simulink library "pm_machines_library"  (R2016b)
settings: Solver=ode45  StartTime=0.0  StopTime=10.0  RelTol=1e-3  EnableMultiTasking=on
libraries: powerlib x9, pm_machines_library x4, powerlib_extras x3
settings Model: Creator=s0237326  LastModifiedBy=rcrozier
settings DataIOCC: LimitDataPoints=on  SaveFormat=Array  SignalLoggingSaveFormat=ModelDataLogs
settings OptimizationCC: ExpressionDepthLimit=2147483647  LifeSpan=inf
settings DebuggingCC: UnderspecifiedInitializationDetection=Classic  MergeDetectMultiDrivingBlocksExec=none  SolverPrmCheckMsg=warning  FcnCallInpInsideContextMsg=warning  StateNameClashWarn=warning  SFUnexpectedBacktrackingDiag=warning  SFNoUnconditionalDefaultTransitionDiag=warning  SFExecutionAtInitializationDiag=none
settings HardwareCC: ProdBitPerPointer=32  ProdBitPerSizeT=32  ProdBitPerPtrDiffT=32  ProdLargestAtomicFloat=None  ProdIntDivRoundTo=Undefined  ProdEndianess=Unspecified  ProdWordSize=32  ProdHWDeviceType=32-bit Generic
settings ModelReferenceCC: PropagateSignalLabelsOutOfModel=off
settings GRTTargetCC: TargetLangStandard=C89/C90 (ANSI)  GeneratePreprocessorConditionals=Disable all  CombineOutputUpdateFcns=off  GRTInterface=on
settings ConfigComp: CovMetricSettings=dw  CovHtmlReporting=on  CovSaveCumulativeToWorkspaceVar=on  CovSaveSingleToWorkspaceVar=on  CovExternalEMLEnable=off

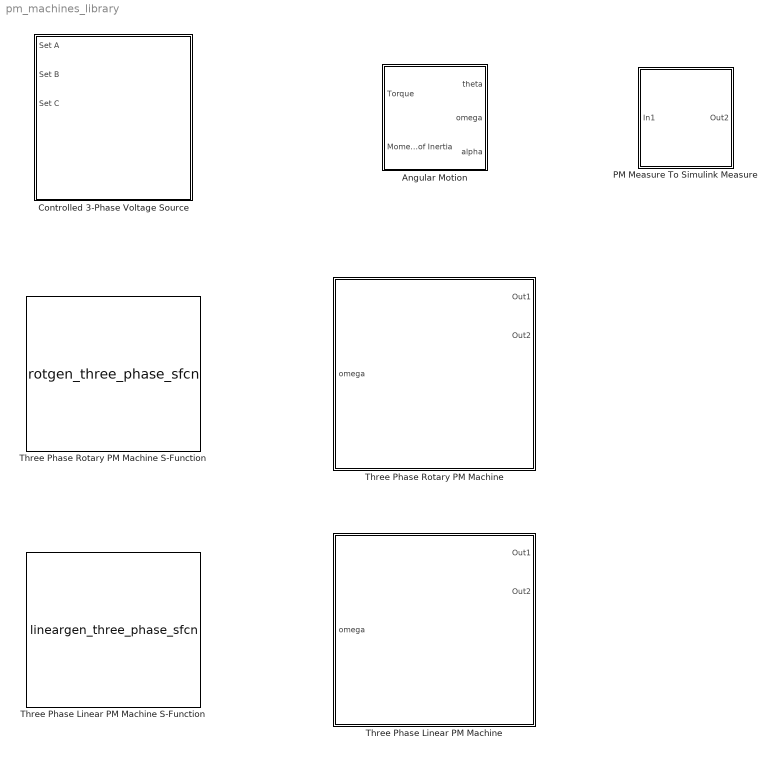
== system pm_machines_library ==
  Angular Motion : Subsystem
  Controlled 3-Phase Voltage Source : Subsystem  mask(Controlled 3-Phase Voltage Source){}
      mask help: Controlled 3-Phase Voltage Source Mask
      mask DialogControl DescGroupVar Prompt: Controlled Three Phase Voltage Source
      mask DialogControl DescTextVar Prompt: A block of three SimPowerSystems controlled voltage sources for interfacing non-SimPowerSystems three phase signals into SimPowerSystems simulations. Provided for convenience, used by other library blocks.
  PM Measure To Simulink Measure : Subsystem  mask{ref_type=Stationary}
      mask prompts: ref_type "dq Reference Type"
      mask TypeOptions ref_type: Synchronous | Stationary
      mask DialogControl DescTextVar Prompt: Converts the outputs of the PM Machines library blocks to the same format as the native simulink electrical machine models proide as 'measurements'.
  Three Phase Linear PM Machine : Subsystem  mask{design_data_type_popup=From File, file_name_edit=Enter file path here, design_workspace_edit=[], simoptions_workspace_edit=[]}
      mask prompts: design_data_type_popup "Design Data Type"; file_name_edit "File containing design and Simoptions data structures"; design_workspace_edit "Design structure variable in workspace"; simoptions_workspace_edit "Simoptions structure variable name"
      mask init:
      | data_ready = false;
      | 
      | if design_data_type_popup == 1
      |     
      |     if ~(strcmp(file_name_edit, 'Enter file path here') ...
      |             || isempty(file_name_edit))
      | 
      |         % get the file name
      |         design_data_file = file_name_edit;
      |         
      |         % check it exists
      |         if exist (design_data_file, 'file') == 2
      |             % check if right data is in file
      |             try
      |                 load (design_data_file, 'design', 'simoptions');
      |             catch ME
      |                 error ('RENEWNET:rotgen_three_phase_sfcn:badfile', ...
      |                 'Loading design data from file\n\n %s\n\nfailed with the following error message:\n\n"%s"\n\n', ...
      |                     design_data_file, ME.message);
      |             end
      |             
      |             data_ready = true;
      | 
      |         else
      |             error ('RENEWNET:rotgen_three_phase_sfcn:badfile', ...
      |                 'Design data file\n: %s\ndoes not appear to exist', design_data_file);
      |         end
      |     
      |     end
      | 
      | elseif design_data_type_popup == 2
      |     % get the variable names
      |     design = design_workspace_edit;
      |     simoptions = simoptions_workspace_edit;
      |     
      |     if ~isempty (design) && ~isempty (simoptions)
      |         data_ready = true;
      |     end
      | else
      |     error ('RENEWNET:rotgen_three_phase_sfcn:baddatatype', ...
      |         'Invalid Data Type popup value')
      | end
      | 
      | if data_ready
      |     
      |     % do some checks on the data
      |     if design.Phases ~= 3
      |         error('Design must have three Phases.')
      |     end
      | 
      |     if ~isfield(design, 'slm_fluxlinkage')
      |         error('Design data does not appear to be complete (no flux linage info)')
      |     end
      | 
      |     blk = gcb;                                         
      |     % set_param([gcb, '/adder1/Gain'],'Gain','A')
      | 
      |     set_param([blk, '/Windings'], 'SelfImpedance1', sprintf('[%f %f]', design.PhaseResistance(1), design.PhaseInductance(1)));
      |     set_param([blk, '/Windings'], 'SelfImpedance2', sprintf('[%f %f]', design.PhaseResistance(2), design.PhaseInductance(1)));
      |     set_param([blk, '/Windings'], 'SelfImpedance3', sprintf('[%f %f]', design.PhaseResistance(3), design.PhaseInductance(1)));
      | 
      |     if numel(design.PhaseInductance) == 2
      |         set_param([blk, '/Windings'], 'MutualImpedance', sprintf('[0 %f]', design.PhaseInductance(2)));
      |     else
      |         set_param([blk, '/Windings'], 'MutualImpedance', '[0 0]');
      |     end
      |     
      |     % put the data into UserData for the block
      |     set_param([blk, '/Three Phase Rotary PM Machine S-Function'], ...
      |         'UserData', struct ('design', design, ...
      |                             'simoptions', simoptions, ...
      |                             'data_ready', true));
      | 
      | end
      mask TypeOptions design_data_type_popup: Three Phase Linear PM Machine S-Function/design_data_type_popup
      mask Callback design_data_type_popup:
      | blk = gcb;
      | 
      | % Get the mask parameter values. This is a cell
      | %   array of character vectors.
      | maskStr = get_param(blk,'design_data_type_popup');
      | 
      | % The pop-up menu is the first mask parameter.
      | %   Check the value selected in the pop-up
      | if strcmp(maskStr,'From File')
      | 
      |     % Make file name box visible only
      |     set_param(gcb,'MaskEnables',{'on';'on';'off';'off'});
      | 
      | else
      | 
      |     % Make variable name boxes visible only
      |     set_param(gcb,'MaskEnables',{'on';'off';'on';'on'});
      | 
      |     % Set the character vector in the Values field equal to the
      |     % character vector selected in the Gain pop-up menu.
      | 
      | %     %maskStr{2}=maskStr{1};
      | %     set_param(gcb,'editvalue',maskStr);
      | 
      | end
      mask TypeOptions file_name_edit: Three Phase Linear PM Machine S-Function/file_name_edit
      mask TypeOptions design_workspace_edit: Three Phase Linear PM Machine S-Function/design_workspace_edit
      mask TypeOptions simoptions_workspace_edit: Three Phase Linear PM Machine S-Function/simoptions_workspace_edit
      mask DialogControl DescTextVar Prompt: Three phase linear permanent magnet machine.
      mask Display:
      | port_label('input', 1, 'Velocity')
      | port_label('output', 1, 'Force')
      | port_label('output', 2, 'Meas')
      | port_label('rconn', 1, 'Phase A')
      | port_label('rconn', 2, 'Phase B')
      | port_label('rconn', 3, 'Phase C')
  Three Phase Linear PM Machine S-Function : M-S-Function  FunctionName=lineargen_three_phase_sfcn  Parameters=design_data_type_popup, file_name_edit, design_workspace_edit, simoptions_workspace_edit  mask{design_data_type_popup=From File, file_name_edit=Enter file path here, design_workspace_edit=[], simoptions_workspace_edit=[]}
      mask prompts: design_data_type_popup "Design Data Type"; file_name_edit "File containing design and Simoptions data structures"; design_workspace_edit "Design structure variable in workspace"; simoptions_workspace_edit "Simoptions structure variable name"
      mask TypeOptions design_data_type_popup: From File | From Workspace
      mask Callback design_data_type_popup:
      | blk = gcb;
      | 
      | % Get the mask parameter values. This is a cell
      | %   array of character vectors.
      | maskStr = get_param(blk,'design_data_type_popup');
      | 
      | % The pop-up menu is the first mask parameter.
      | %   Check the value selected in the pop-up
      | if strcmp(maskStr,'From File')
      | 
      |     % Make file name box visible only
      |     set_param(gcb,'MaskEnables',{'on';'on';'off';'off'});
      | 
      | else
      | 
      |     % Make variable name boxes visible only
      |     set_param(gcb,'MaskEnables',{'on';'off';'on';'on'});
      | 
      |     % Set the character vector in the Values field equal to the
      |     % character vector selected in the Gain pop-up menu.
      | 
      | %     %maskStr{2}=maskStr{1};
      | %     set_param(gcb,'editvalue',maskStr);
      | 
      | end
      mask DialogControl DescTextVar Prompt: Block for simulation of a three phase linear permanent magnet machine based on a Level-2 S-Function. This is a low level block, used in the higher-level 'Three Phase Linear PM Machine' block which is intended for users. You may want to use this if you do not wish to use SimPowerSystems components.
      mask Display:
      | port_label('input', 1, 'displacement')
      | port_label('input', 2, 'velocity')
      | port_label('input', 3, 'Phase A Current')
      | port_label('input', 4, 'Phase B Current')
      | port_label('input', 5, 'Phase C Current')
      | port_label('output', 1, 'Force')
      | port_label('output', 2, 'Phase A EMF')
      | port_label('output', 3, 'Phase B EMF')
      | port_label('output', 4, 'Phase C EMF')
      | port_label('output', 5, 'Meas')
  Three Phase Rotary PM Machine : Subsystem  mask{design_data_type_popup=From File, file_name_edit=Enter file path here, design_workspace_edit=[], simoptions_workspace_edit=[]}
      mask prompts: design_data_type_popup "Design Data Type"; file_name_edit "File containing design and Simoptions data structures"; design_workspace_edit "Design structure variable in workspace"; simoptions_workspace_edit "Simoptions structure variable name"
      mask init: same as pm_machines_library/Three Phase Linear PM Machine
      mask TypeOptions design_data_type_popup: Three Phase Rotary PM Machine S-Function/design_data_type_popup
      mask Callback design_data_type_popup:
      | blk = gcb;
      | 
      | % Get the mask parameter values. This is a cell
      | %   array of character vectors.
      | maskStr = get_param(blk,'design_data_type_popup');
      | 
      | % The pop-up menu is the first mask parameter.
      | %   Check the value selected in the pop-up
      | if strcmp(maskStr,'From File')
      | 
      |     % Make file name box visible only
      |     set_param(gcb,'MaskEnables',{'on';'on';'off';'off'});
      | 
      | else
      | 
      |     % Make variable name boxes visible only
      |     set_param(gcb,'MaskEnables',{'on';'off';'on';'on'});
      | 
      |     % Set the character vector in the Values field equal to the
      |     % character vector selected in the Gain pop-up menu.
      | 
      | %     %maskStr{2}=maskStr{1};
      | %     set_param(gcb,'editvalue',maskStr);
      | 
      | end
      mask TypeOptions file_name_edit: Three Phase Rotary PM Machine S-Function/file_name_edit
      mask TypeOptions design_workspace_edit: Three Phase Rotary PM Machine S-Function/design_workspace_edit
      mask TypeOptions simoptions_workspace_edit: Three Phase Rotary PM Machine S-Function/simoptions_workspace_edit
      mask DialogControl DescTextVar Prompt: Three phase rotary permanent magnet machine.
      mask Display:
      | port_label('input', 1, 'Omega')
      | port_label('output', 1, 'Torque')
      | port_label('output', 2, 'Meas')
      | port_label('rconn', 1, 'Phase A')
      | port_label('rconn', 2, 'Phase B')
      | port_label('rconn', 3, 'Phase C')
  Three Phase Rotary PM Machine S-Function : M-S-Function  FunctionName=rotgen_three_phase_sfcn  Parameters=design_data_type_popup, file_name_edit, design_workspace_edit, simoptions_workspace_edit  mask{design_data_type_popup=From FIle, file_name_edit=Enter file path here, design_workspace_edit=[], simoptions_workspace_edit=[]}
      mask prompts: design_data_type_popup "Design Data Type"; file_name_edit "File containing design and Simoptions data structures"; design_workspace_edit "Design structure variable in workspace"; simoptions_workspace_edit "Simoptions structure variable name"
      mask TypeOptions design_data_type_popup: From File | From Workspace
      mask Callback design_data_type_popup:
      | blk = gcb;
      | 
      | % Get the mask parameter values. This is a cell
      | %   array of character vectors.
      | maskStr = get_param(blk,'design_data_type_popup');
      | 
      | % The pop-up menu is the first mask parameter.
      | %   Check the value selected in the pop-up
      | if strcmp(maskStr,'From File')
      | 
      |     % Make file name box visible only
      |     set_param(gcb,'MaskEnables',{'on';'on';'off';'off'});
      | 
      | else
      | 
      |     % Make variable name boxes visible only
      |     set_param(gcb,'MaskEnables',{'on';'off';'on';'on'});
      | 
      |     % Set the character vector in the Values field equal to the
      |     % character vector selected in the Gain pop-up menu.
      | 
      | %     %maskStr{2}=maskStr{1};
      | %     set_param(gcb,'editvalue',maskStr);
      | 
      | end
      mask DialogControl DescTextVar Prompt: Block for simulation of a three phase rotary permanent magnet machine based on a Level-2 S-Function. This is a low level block, used in the higher-level 'Three Phase Rotary PM Machine' block which is intended for users. You may want to use this if you do not wish to use SimPowerSystems components.
      mask Display:
      | port_label('input', 1, 'theta')
      | port_label('input', 2, 'omega')
      | port_label('input', 3, 'Phase A Current')
      | port_label('input', 4, 'Phase B Current')
      | port_label('input', 5, 'Phase C Current')
      | port_label('output', 1, 'Torque')
      | port_label('output', 2, 'Phase A EMF')
      | port_label('output', 3, 'Phase B EMF')
      | port_label('output', 4, 'Phase C EMF')
      | port_label('output', 5, 'Meas')

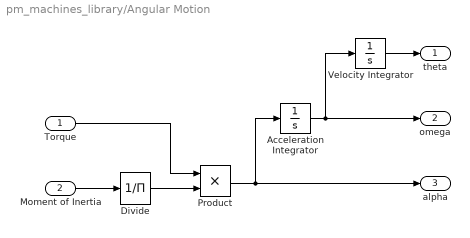
== system pm_machines_library/Angular Motion ==
  Torque : Inport
  Moment of Inertia : Inport  Port=2
  Acceleration Integrator : Integrator
  Divide : Product  Inputs=/
  Product : Product  RndMeth=Zero
  Velocity Integrator : Integrator
  theta : Outport
  omega : Outport  Port=2
  alpha : Outport  Port=3
  wires:
  Product/1 -> alpha/1, Acceleration Integrator/1
  Velocity Integrator/1 -> theta/1
  Acceleration Integrator/1 -> omega/1, Velocity Integrator/1
  Torque/1 -> Product/1
  Moment of Inertia/1 -> Divide/1
  Divide/1 -> Product/2

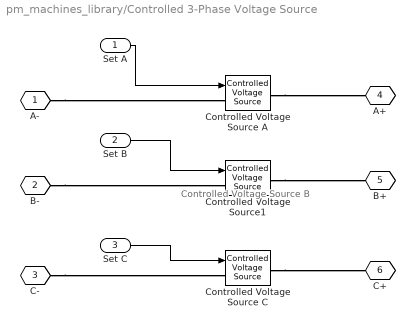
== system pm_machines_library/Controlled 3-Phase Voltage Source ==
  note: Controlled Voltage Source B
  Set A : Inport  PortDimensions=1
  Set B : Inport  Port=2  PortDimensions=1
  Set C : Inport  Port=3  PortDimensions=1
  Controlled Voltage Source A : powerlib/Electrical Sources/Controlled Voltage Source  Initialize=off  Source_Type=AC  Amplitude=0  Phase=0  Frequency=0  Measurements=None
  Controlled Voltage Source C : powerlib/Electrical Sources/Controlled Voltage Source  Initialize=off  Source_Type=AC  Amplitude=0  Phase=0  Frequency=0  Measurements=None
  Controlled Voltage Source1 : powerlib/Electrical Sources/Controlled Voltage Source  Initialize=off  Source_Type=AC  Amplitude=0  Phase=0  Frequency=0  Measurements=None
  A- : PMIOPort  Tag=PMCPort  Port=1  Side=Left
  B- : PMIOPort  Tag=PMCPort  Port=2  Side=Left
  C- : PMIOPort  Tag=PMCPort  Port=3  Side=Left
  A+ : PMIOPort  Tag=PMCPort  Port=4  Side=Right
  B+ : PMIOPort  Tag=PMCPort  Port=5  Side=Right
  C+ : PMIOPort  Tag=PMCPort  Port=6  Side=Right
  wires:
  Set C/1 -> Controlled Voltage Source C/1
  Set B/1 -> Controlled Voltage Source1/1
  Set A/1 -> Controlled Voltage Source A/1
  connections:
  A-/RConn1 -- Controlled Voltage Source A/LConn1
  Controlled Voltage Source A/RConn1 -- A+/RConn1
  C-/RConn1 -- Controlled Voltage Source C/LConn1
  Controlled Voltage Source C/RConn1 -- C+/RConn1
  B-/RConn1 -- Controlled Voltage Source1/LConn1
  Controlled Voltage Source1/RConn1 -- B+/RConn1

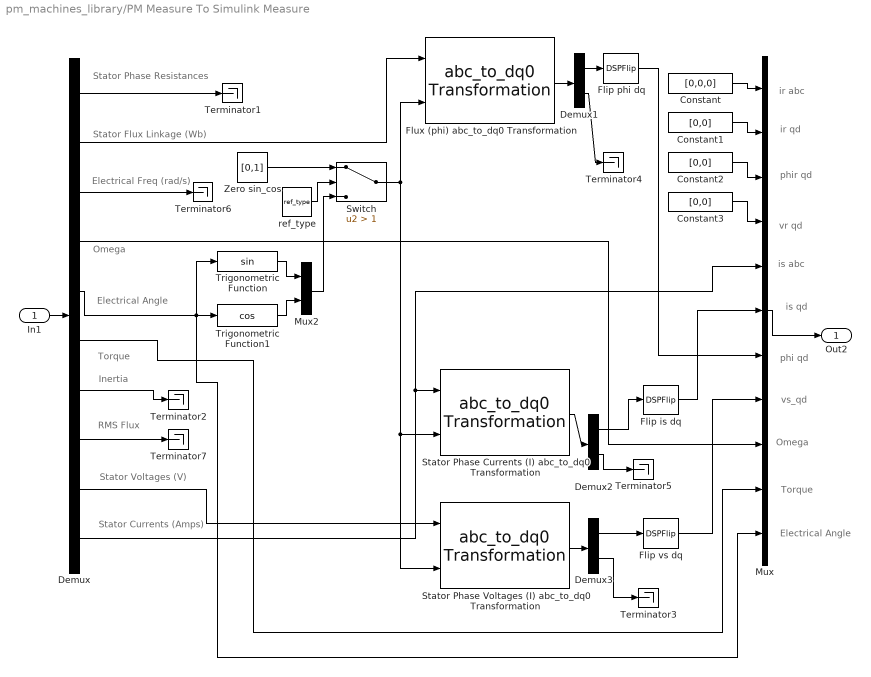
== system pm_machines_library/PM Measure To Simulink Measure ==
  note: RMS Flux
  note: Electrical Freq (rad/s)
  note: Stator Flux Linkage (Wb)
  note: Stator Currents (Amps)
  note: Stator Voltages (V)
  note: Omega
  note: Electrical Angle
  note: Torque
  note: Torque
  note: Omega
  note: vs_qd
  note: is qd
  note: phi qd
  note: is abc
  note: ir abc
  note: ir qd
  note: phir qd
  note: vr qd
  note: Stator Phase Resistances
  note: Inertia
  note: Electrical Angle
  In1 : Inport
  Constant : Constant  Value=[0,0,0]
  Constant1 : Constant  Value=[0,0]
  Constant2 : Constant  Value=[0,0]
  Constant3 : Constant  Value=[0,0]
  Demux : Demux  Outputs=[3, 3, 1, 1, 1, 1, 1, 1, 3, 3]
  Demux1 : Demux  Outputs=[2,1]
  Demux2 : Demux  Outputs=[2,1]
  Demux3 : Demux  Outputs=[2,1]
  Flip is dq : DSPFlip
  Flip phi dq : DSPFlip
  Flip vs dq : DSPFlip
  Flux (phi) abc_to_dq0 Transformation : powerlib_extras/Measurements/abc_to_dq0 Transformation
  Mux : Mux  Inputs=11
  Mux2 : Mux  Inputs=2
  Stator Phase Currents (I) abc_to_dq0 Transformation : powerlib_extras/Measurements/abc_to_dq0 Transformation
  Stator Phase Voltages (I) abc_to_dq0 Transformation : powerlib_extras/Measurements/abc_to_dq0 Transformation
  Switch : Switch  Criteria=u2 > Threshold  Threshold=1  ZeroCross=off
  Terminator{1..7} (7 alike) : Terminator
  Trigonometric Function : Trigonometry
  Trigonometric Function1 : Trigonometry  Operator=cos
  Zero sin_cos : Constant  Value=[0,1]
  ref_type : Constant  Value=ref_type
  Out2 : Outport
  wires:
  Demux/2 -> Flux (phi) abc_to_dq0 Transformation/1
  In1/1 -> Demux/1
  Demux/4 -> Mux/9
  Demux/6 -> Mux/10
  Mux/1 -> Out2/1
  Demux/1 -> Terminator1/1
  Demux/9 -> Stator Phase Voltages (I) abc_to_dq0 Transformation/1
  Demux/10 -> Stator Phase Currents (I) abc_to_dq0 Transformation/1, Mux/5
  Demux/7 -> Terminator2/1
  Demux/5 -> Mux/11, Trigonometric Function/1, Trigonometric Function1/1
  Trigonometric Function/1 -> Mux2/1
  Trigonometric Function1/1 -> Mux2/2
  Flux (phi) abc_to_dq0 Transformation/1 -> Demux1/1
  Stator Phase Currents (I) abc_to_dq0 Transformation/1 -> Demux2/1
  Stator Phase Voltages (I) abc_to_dq0 Transformation/1 -> Demux3/1
  Constant/1 -> Mux/1
  Constant3/1 -> Mux/4
  Constant2/1 -> Mux/3
  Constant1/1 -> Mux/2
  Flip is dq/1 -> Mux/6
  Demux2/1 -> Flip is dq/1
  Demux3/1 -> Flip vs dq/1
  Flip vs dq/1 -> Mux/8
  Demux1/1 -> Flip phi dq/1
  Flip phi dq/1 -> Mux/7
  Demux3/2 -> Terminator3/1
  Demux1/2 -> Terminator4/1
  Demux2/2 -> Terminator5/1
  Demux/3 -> Terminator6/1
  Zero sin_cos/1 -> Switch/1
  Mux2/1 -> Switch/3
  ref_type/1 -> Switch/2
  Switch/1 -> Stator Phase Currents (I) abc_to_dq0 Transformation/2, Stator Phase Voltages (I) abc_to_dq0 Transformation/2, Flux (phi) abc_to_dq0 Transformation/2
  Demux/8 -> Terminator7/1

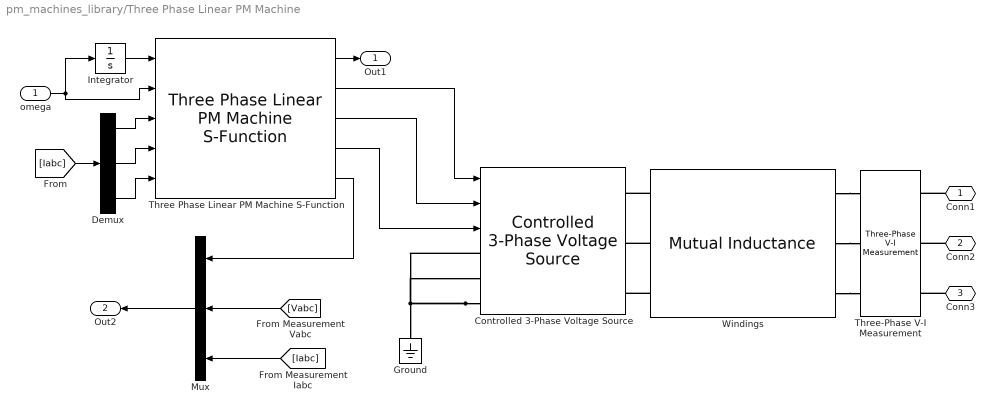
== system pm_machines_library/Three Phase Linear PM Machine ==
  omega : Inport
  Controlled 3-Phase Voltage Source : pm_machines_library/Controlled 3-Phase Voltage Source
  Demux : Demux  Outputs=3
  Ground : powerlib/Elements/Ground  LConnTagsString=a
  Integrator : Integrator
  Mux : Mux  Inputs=3
  Three Phase Linear PM Machine S-Function : pm_machines_library/Three Phase Linear PM Machine S-Function  design_data_type_popup=From File  file_name_edit=Enter file path here  design_workspace_edit=design_workspace_edit  simoptions_workspace_edit=simoptions_workspace_edit
  Three-Phase V-I Measurement : powerlib/Measurements/Three-Phase V-I Measurement  VoltageMeasurement=phase-to-ground  SetLabelV=on  LabelV=Vabc  Vpu=off  VpuLL=off  CurrentMeasurement=yes  SetLabelI=on  LabelI=Iabc  Ipu=off  Pbase=100e6  Vbase=500e3  OutputType=Complex  PhasorSimulation=off  PSBequivalent=0
  Windings : powerlib/Elements/Mutual Inductance  LConnTagsString=a|b|c  RConnTagsString=A|B|C  TypeOfMutual=Two or three windings with equal mutual terms  NumberOfWindings=3  SelfImpedance1=[218.993012 0.000104]  SelfImpedance2=[218.993012 0.000104]  ThreeWindings=on  SelfImpedance3=[218.993012 0.000104]  MutualImpedance=[0 0.000000]  InductanceMatrix="[1.0 0.9  0.9 ;  0.9 1.0  0.9;  0.9 0.9 1.0 ] * 1e-3"  ResistanceMatrix="[1.0 0.9  0.9 ;  0.9 1.0  0.9;  0.9 0.9 1.0 ]"  Measurements=None
      settings: AttributesFormatString=\n
  Conn1 : PMIOPort  Port=1  Side=Right
  Conn2 : PMIOPort  Port=2  Side=Right
  Conn3 : PMIOPort  Port=3  Side=Right
  Out1 : Outport
  Out2 : Outport  Port=2
  wires:
  Demux/3 -> Three Phase Linear PM Machine S-Function/5
  Demux/2 -> Three Phase Linear PM Machine S-Function/4
  Demux/1 -> Three Phase Linear PM Machine S-Function/3
  [Iabc] -> Demux/1
  Three Phase Linear PM Machine S-Function/4 -> Controlled 3-Phase Voltage Source/3
  Three Phase Linear PM Machine S-Function/3 -> Controlled 3-Phase Voltage Source/2
  Three Phase Linear PM Machine S-Function/2 -> Controlled 3-Phase Voltage Source/1
  Integrator/1 -> Three Phase Linear PM Machine S-Function/1
  omega/1 -> Three Phase Linear PM Machine S-Function/2, Integrator/1
  Three Phase Linear PM Machine S-Function/1 -> Out1/1
  Three Phase Linear PM Machine S-Function/5 -> Mux/1
  [Vabc] -> Mux/2
  [Iabc] -> Mux/3
  Mux/1 -> Out2/1
  connections:
  Controlled 3-Phase Voltage Source/LConn3 -- Controlled 3-Phase Voltage Source/LConn2 -- Controlled 3-Phase Voltage Source/LConn1 -- Ground/LConn1
  Windings/LConn1 -- Controlled 3-Phase Voltage Source/RConn1
  Windings/LConn2 -- Controlled 3-Phase Voltage Source/RConn2
  Windings/LConn3 -- Controlled 3-Phase Voltage Source/RConn3
  Windings/RConn1 -- Three-Phase V-I Measurement/LConn1
  Windings/RConn2 -- Three-Phase V-I Measurement/LConn2
  Windings/RConn3 -- Three-Phase V-I Measurement/LConn3
  Conn1/RConn1 -- Three-Phase V-I Measurement/RConn1
  Conn2/RConn1 -- Three-Phase V-I Measurement/RConn2
  Conn3/RConn1 -- Three-Phase V-I Measurement/RConn3

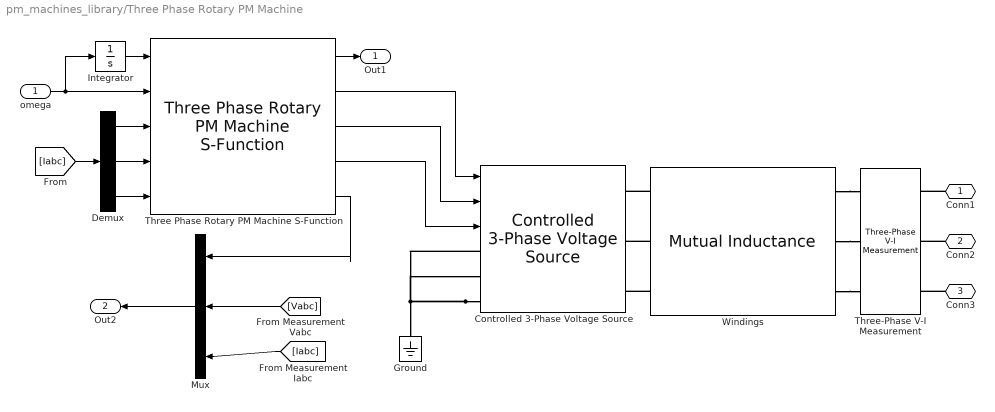
== system pm_machines_library/Three Phase Rotary PM Machine ==
  omega : Inport
  Controlled 3-Phase Voltage Source : pm_machines_library/Controlled 3-Phase Voltage Source
  Demux : Demux  Outputs=3
  Ground : powerlib/Elements/Ground  LConnTagsString=a
  Integrator : Integrator
  Mux : Mux  Inputs=3
  Three Phase Rotary PM Machine S-Function : pm_machines_library/Three Phase Rotary PM Machine S-Function  design_data_type_popup=From File  file_name_edit=Enter file path here  design_workspace_edit=design_workspace_edit  simoptions_workspace_edit=simoptions_workspace_edit
  Three-Phase V-I Measurement : powerlib/Measurements/Three-Phase V-I Measurement  VoltageMeasurement=phase-to-ground  SetLabelV=on  LabelV=Vabc  Vpu=off  VpuLL=off  CurrentMeasurement=yes  SetLabelI=on  LabelI=Iabc  Ipu=off  Pbase=100e6  Vbase=500e3  OutputType=Complex  PhasorSimulation=off  PSBequivalent=0
  Windings : powerlib/Elements/Mutual Inductance  LConnTagsString=a|b|c  RConnTagsString=A|B|C  TypeOfMutual=Two or three windings with equal mutual terms  NumberOfWindings=3  SelfImpedance1=[218.993012 0.000104]  SelfImpedance2=[218.993012 0.000104]  ThreeWindings=on  SelfImpedance3=[218.993012 0.000104]  MutualImpedance=[0 0.000000]  InductanceMatrix="[1.0 0.9  0.9 ;  0.9 1.0  0.9;  0.9 0.9 1.0 ] * 1e-3"  ResistanceMatrix="[1.0 0.9  0.9 ;  0.9 1.0  0.9;  0.9 0.9 1.0 ]"  Measurements=None
      settings: AttributesFormatString=\n
  Conn1 : PMIOPort  Port=1  Side=Right
  Conn2 : PMIOPort  Port=2  Side=Right
  Conn3 : PMIOPort  Port=3  Side=Right
  Out1 : Outport
  Out2 : Outport  Port=2
  wires:
  Demux/3 -> Three Phase Rotary PM Machine S-Function/5
  Demux/2 -> Three Phase Rotary PM Machine S-Function/4
  Demux/1 -> Three Phase Rotary PM Machine S-Function/3
  [Iabc] -> Demux/1
  Three Phase Rotary PM Machine S-Function/4 -> Controlled 3-Phase Voltage Source/3
  Three Phase Rotary PM Machine S-Function/3 -> Controlled 3-Phase Voltage Source/2
  Three Phase Rotary PM Machine S-Function/2 -> Controlled 3-Phase Voltage Source/1
  Integrator/1 -> Three Phase Rotary PM Machine S-Function/1
  omega/1 -> Three Phase Rotary PM Machine S-Function/2, Integrator/1
  Three Phase Rotary PM Machine S-Function/1 -> Out1/1
  Three Phase Rotary PM Machine S-Function/5 -> Mux/1
  [Vabc] -> Mux/2
  [Iabc] -> Mux/3
  Mux/1 -> Out2/1
  connections:
  Controlled 3-Phase Voltage Source/LConn3 -- Controlled 3-Phase Voltage Source/LConn2 -- Controlled 3-Phase Voltage Source/LConn1 -- Ground/LConn1
  Windings/LConn1 -- Controlled 3-Phase Voltage Source/RConn1
  Windings/LConn2 -- Controlled 3-Phase Voltage Source/RConn2
  Windings/LConn3 -- Controlled 3-Phase Voltage Source/RConn3
  Windings/RConn1 -- Three-Phase V-I Measurement/LConn1
  Windings/RConn2 -- Three-Phase V-I Measurement/LConn2
  Windings/RConn3 -- Three-Phase V-I Measurement/LConn3
  Conn1/RConn1 -- Three-Phase V-I Measurement/RConn1
  Conn2/RConn1 -- Three-Phase V-I Measurement/RConn2
  Conn3/RConn1 -- Three-Phase V-I Measurement/RConn3
